simulink model "fxpdemo_feedback"  (Simulink 6.0)
settings: Solver=ode4  SolverMode=SingleTasking  StartTime=0.0  StopTime=4-2*tsamp  FixedStep=tsamp  RelTol=1e-3  AbsTol=1e-6
PreLoadFcn:
  | preload_feedback
values from neighbouring files (symbols this model uses):
  dden = [ ... (first row only)    [preload_feedback.m]
  pden = conv( pden, [ 1/wn 1 ] )    [preload_feedback.m]
  pnum = 4 * wn^2    (= 1600)    [preload_feedback.m]
  tsamp = 0.01    [preload_feedback.m]
libraries: fixpt_lib_4 x4, fixpt_lib_3p1 x1
settings Model: RequirementInfo=9  CovMetricSettings=d  MinMaxOverflowLogging=MinMaxAndOverflow  Creator=andyb  LastModifiedBy=andyb  ExtModeTrigMode=oneshot  ExtModeArmWhenConnect=off  ExtModeAutoUpdateStatusClock=off  LimitDataPoints=off  IntegerOverflowMsg=none  ParameterDowncastMsg=warning  ParameterOverflowMsg=warning  ParameterPrecisionLossMsg=none  RTWInlineParameters=on  BooleanDataType=on  ZeroCrossControl=UseLocalSettings  ProdHWDeviceType=Microprocessor  TargetHWChar=2  TargetHWWordLengths=8,16,32,32  RTWMathFcnLibMatFile=iso_c_tmw.mat  RTWOptions="-aEnforceIntegerDowncast=1 -aFoldNonRolledExpr=1 -aInlineInvariantSignals=1 -aInlineParameters=1 -aLocalBlockOutputs=1 -aRollThreshold=5 -aGenerateReport=1 -aGenCodeOnly=0 -aRTWVerbose=1 -aForceParamTrailComments=0 -aGenerateComments=0 -aIgnoreCustomStorageClasses=1 -aIncHierarchyInIds=0 -aMaxRTWIdLen=31 -aShowEliminatedStatements=0 -aPrefixModelToSubsysFcnNames=1 -aIncDataTypeInIds=1 -aInlinedPrmAccess=\"Literals\" -aTargetFcnLib=\"iso_c_tmw.mat\" -aGenerateFullHeader=1 -aIsPILTarget=0 -aExtMode=0 -aExtModeStaticAlloc=0 -aExtModeTesting=0 -aExtModeStaticAllocSize=1000000 -aExtModeTransport=0 -aLogVarNameModifier=\"rt_\" -aRTWCAPISignals=0 -aRTWCAPIParams=0"
settings DataIOCC: LimitDataPoints=off  SignalLoggingName=sigsOut
settings OptimizationCC: InlineParams=on  MultiInstanced=off
settings FormatCC: IgnoreBidirectionalLines=off
settings DebuggingCC: IntegerOverflowMsg=none  ParameterDowncastMsg=warning  ParameterOverflowMsg=warning  ParameterPrecisionLossMsg=none
settings HardwareCC: ProdHWDeviceType=Microprocessor  ShiftRightIntArith=on  TargetHWCharacteristics=InheritFromRTWHook
settings RTWCC: GenerateReport=on
settings CodeAppCC: GenerateComments=off  FileBanners=off  IncDataTypeInIds=on
settings GRTTargetCC: TargetFcnLib=iso_c_tmw.mat  IsERTTarget=off

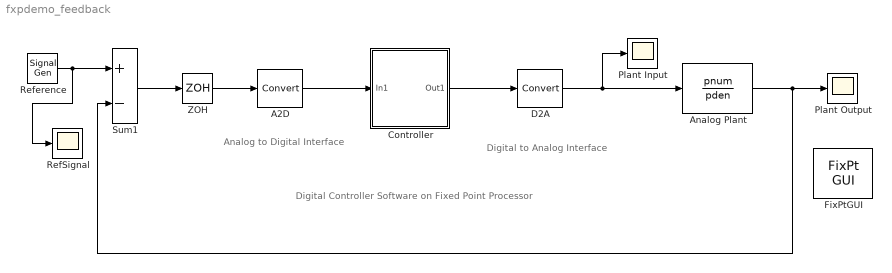
== system fxpdemo_feedback ==
  note: Analog to Digital
      | Interface
  note: Digital Controller
      | Software on
      | Fixed Point
      | Processor
  note: Digital to Analog
      | Interface
  A2D : DataTypeConversion  OutDataTypeMode=Specify via dialog  OutDataType=sfix(8)  OutScaling=2^-4  RndMeth=Nearest  SaturateOnIntegerOverflow=on  LockScale=on
  Analog Plant : TransferFcn  Numerator=pnum  Denominator=pden
  Controller : Subsystem
  D2A : DataTypeConversion  OutDataTypeMode=double
  FixPtGUI : fixpt_lib_3p1/FixPt GUI
  Plant Input : Scope
      settings: TickLabels=on  SaveName=PlantInput
  Plant Output : Scope
      settings: TickLabels=on  YMin=-4  YMax=2.5  SaveName=PlantOutput
  RefSignal : Scope
      settings: TickLabels=on  TimeRange=4  YMin=-2  YMax=2  SaveName=ReferenceSignal
  Reference : SignalGenerator  WaveForm=square  Amplitude=2  Frequency=0.25
  Sum1 : Sum  Inputs=+-  SaturateOnIntegerOverflow=on  InputSameDT=on
  ZOH : ZeroOrderHold  SampleTime=tsamp
  wires:
  A2D/1 -> Controller/1(In1)
  Controller/1(Out1) -> D2A/1
  ZOH/1 -> A2D/1
  Reference/1 -> RefSignal/1, Sum1/1
  D2A/1 -> Analog Plant/1, Plant Input/1
  Analog Plant/1 -> Plant Output/1, Sum1/2
  Sum1/1 -> ZOH/1

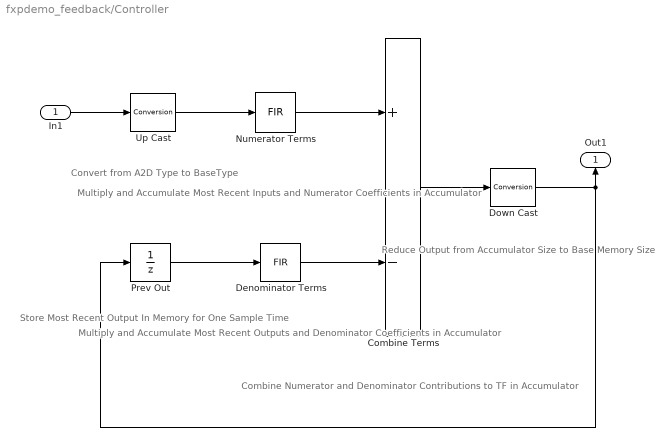
== system fxpdemo_feedback/Controller ==
  note: Convert from
      | A2D Type
      | to BaseType
  note: Multiply and Accumulate
      | Most Recent Inputs and
      | Numerator Coefficients
      | in Accumulator
  note: Multiply and Accumulate
      | Most Recent Outputs and
      | Denominator Coefficients
      | in Accumulator
  note: Store Most
      | Recent Output
      | In Memory for
      | One Sample Time
  note: Combine Numerator
      | and Denominator
      | Contributions to TF
      | in Accumulator
  note: Reduce Output from
      | Accumulator Size to
      | Base Memory Size
  In1 : Inport
  Combine Terms : Sum  Inputs=+-  ShowAdditionalParam=on  OutDataTypeMode=Specify via dialog  OutDataType=AccumType  OutScaling=2^(-12)  SaturateOnIntegerOverflow=on
  Denominator Terms : fixpt_lib_4/Filters/FIR  mgainval=dden(2:length(dden))  vinit=0.0  samptime=tsamp  GainDataTypeScalingMode=Specify via dialog  GainDataType=BaseType  GainScaling=2^-14  MatRadixGroup=Best Precision: Element-wise  OutputDataTypeScalingMode=Specify via dialog  OutDataType=AccumType  OutScaling=2^(-12)  DoSatur=on
  Down Cast : fixpt_lib_4/Data Type/Conversion  ConvertRealWorld=Real World Value  OutputDataTypeScalingMode=Specify via dialog  OutDataType=BaseType  OutScaling=2^(-5)  DoSatur=on
  Numerator Terms : fixpt_lib_4/Filters/FIR  mgainval=dnum  vinit=0.0  samptime=tsamp  GainDataTypeScalingMode=Specify via dialog  GainDataType=BaseType  GainScaling=2^-14  MatRadixGroup=Best Precision: Element-wise  OutputDataTypeScalingMode=Specify via dialog  OutDataType=AccumType  OutScaling=2^(-12)  DoSatur=on
  Prev Out : UnitDelay  X0=0.0  SampleTime=tsamp
  Up Cast : fixpt_lib_4/Data Type/Conversion  ConvertRealWorld=Real World Value  OutputDataTypeScalingMode=Specify via dialog  OutDataType=BaseType  OutScaling=2^(-14)  DoSatur=on
  Out1 : Outport  Orientation=up  InitialOutput=0
  wires:
  Combine Terms/1 -> Down Cast/1
  Denominator Terms/1 -> Combine Terms/2
  Numerator Terms/1 -> Combine Terms/1
  Prev Out/1 -> Denominator Terms/1
  Up Cast/1 -> Numerator Terms/1
  In1/1 -> Up Cast/1
  Down Cast/1 -> Prev Out/1, Out1/1
